simulink model "clonado_controlador"  (R2023b)
settings: Solver=ode45  StartTime=0.0  StopTime=10000  RelTol=1e-3
values from neighbouring files (symbols this model uses):
  D = 0    [control_pid_tuning.m]
libraries: neural x25, simulink x2, slpidlib x1
settings Model: Creator=q  LastModifiedBy=q

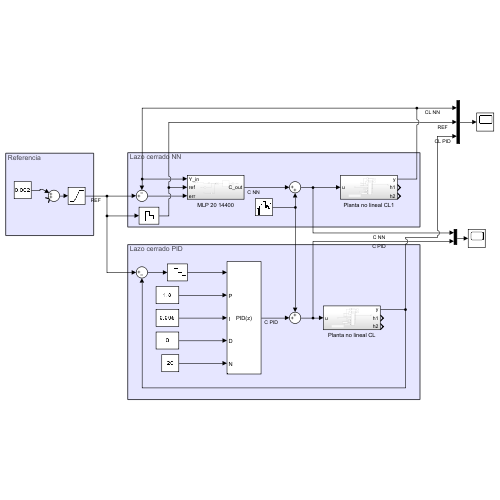
[thumbnail: Simulink's stored preview of the top-level diagram]
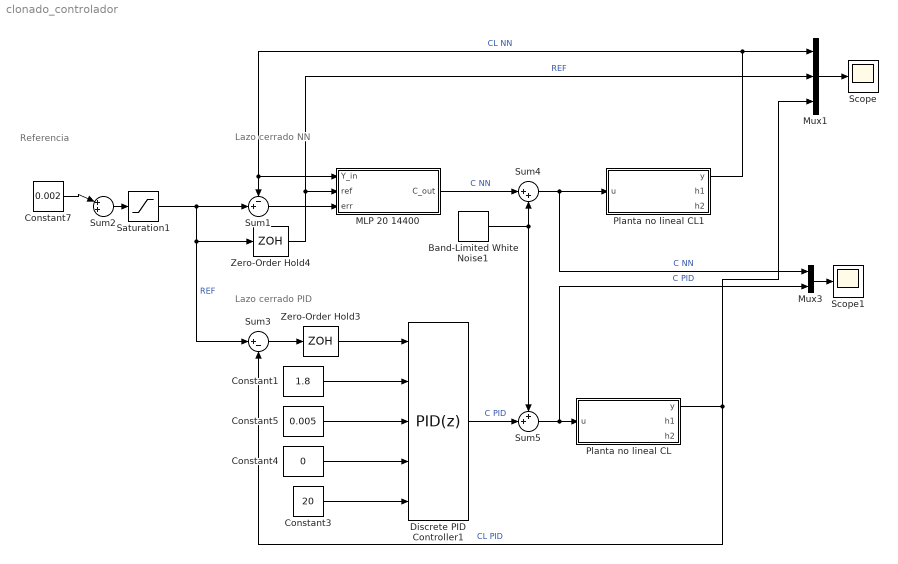
== system clonado_controlador ==
  note: Lazo cerrado NN
  note: Lazo cerrado PID
  note: Referencia
  Band-Limited White Noise1 : simulink/Sources/Band-Limited White Noise  Cov=[0.000002]  Ts=1500  seed=[23341]
  Constant1 : Constant  Value=1.8
  Constant3 : Constant  Value=20
  Constant4 : Constant  Value=0
  Constant5 : Constant  Value=0.005
  Constant7 : Constant  Value=0.002
  Discrete PID Controller1 : slpidlib/PID Controller  Controller=PID  Form=Parallel  TimeDomain=Discrete-time  UseExternalTs=off  SampleTime=-1  IntegratorMethod=Forward Euler  FilterMethod=Forward Euler  ControllerParametersSource=external  P=1  I=1  UseKiTs=off  D=0  N=100  UseFilter=on  TunerSelectOption=Transfer Function Based (PID Tuner App)  InitialConditionSource=internal  InitialConditionForIntegrator=0  InitialConditionForFilter=0  DifferentiatorICPrevScaledInput=0  ExternalReset=none  TrackingMode=off  Kt=1  LimitOutput=off  SatLimitsSource=internal  UpperSaturationLimit=inf  LowerSaturationLimit=-inf  LinearizeAsGain=off  AntiWindupMode=none  Kb=1  LimitIntegrator=off  UpperIntegratorSaturationLimit=inf  LowerIntegratorSaturationLimit=-inf  POutMin=[]  POutMax=[]  IOutMin=[]  IOutMax=[]  DOutMin=[]  DOutMax=[]  NOutMin=[]  NOutMax=[]  SumOutMin=[]  SumOutMax=[]  SaturationOutMin=[]  SaturationOutMax=[]  PParamMin=[]  PParamMax=[]  IParamMin=[]  IParamMax=[]  DParamMin=[]  DParamMax=[]  NParamMin=[]  NParamMax=[]  KbParamMin=[]  KbParamMax=[]  KtParamMin=[]  KtParamMax=[]  KbOutMin=[]  KbOutMax=[]  KtOutMin=[]  KtOutMax=[]  IntegratorOutMin=[]  IntegratorOutMax=[]  FilterOutMin=[]  FilterOutMax=[]  SumI1OutMin=[]  SumI1OutMax=[]  SumI2OutMin=[]  SumI2OutMax=[]  SumI3OutMin=[]  SumI3OutMax=[]  SumI4OutMin=[]  SumI4OutMax=[]  SumDOutMin=[]  SumDOutMax=[]  DifferentiatorOutMin=[]  DifferentiatorOutMax=[]  FilterDiffOutCoefMin=[]  FilterDiffOutCoefMax=[]  ReciprocalOutMin=[]  ReciprocalOutMax=[]  SumDenOutMin=[]  SumDenOutMax=[]  SumNumOutMin=[]  SumNumOutMax=[]  DivideOutMin=[]  DivideOutMax=[]  UdiffTsProdOutMin=[]  UdiffTsProdOutMax=[]  NTsProdOutMin=[]  NTsProdOutMax=[]  UintegralTsProdOutMin=[]  UintegralTsProdOutMax=[]  UngainTsProdOutMin=[]  UngainTsProdOutMax=[]  ClampingZeroOutDataTypeStr=Inherit: Inherit via back propagation  ClampingZeroOutMin=[]  ClampingZeroOutMax=[]  FilterDenConstantOutDataTypeStr=Inherit: Inherit via back propagation  FilterDenConstantOutMin=[]  FilterDenConstantOutMax=[]  PCopyOutDataTypeStr=Inherit: Inherit via back propagation  PCopyOutMin=[]  PCopyOutMax=[]  NCopyOutDataTypeStr=Inherit: Inherit via back propagation  NCopyOutMin=[]  NCopyOutMax=[]  IntegratorContinuousStateAttributes=''  IntegratorStateMustResolveToSignalObject=off  IntegratorRTWStateStorageClass=Auto  FilterContinuousStateAttributes=''  FilterStateMustResolveToSignalObject=off  FilterRTWStateStorageClass=Auto  ParallelPVariant=ExternalParameters  IdealPVariant=Disabled  IVariant=ExternalParameters  DVariant=ExternalParameters  IntegratorVariant=Discrete  SatVariant=Disabled  AWVariant=Passthrough  PCopyVariant=Disabled  TRVariant=Disabled  FdbkBlocksVariant=Forward  IdealPFdbkVariant=Disabled  SatFdbkVariant=Disabled  DerivativeFilterVariant=ForwardEulerFilter  NVariant=ExternalParameters  NCopyVariant=Disabled  FilterICVariant=InternalICsFilter  IntegratorICVariant=InternalICs  ExternalResetVariant=Disabled  TRSumVariant=Passthrough  SumFdbkVariant=Disabled  SumVariant=Sum_PID  TsampFilterVariant=InternalTs  TsampNgainVariant=Passthrough  TsampIntegralVariant=Disabled_SignalSpec  ExternalSaturationOutDataTypeStr=Inherit: Same as second input
      settings: LibrarySourceBlock=simulink/Discrete/Discrete PID Controller
  MLP 20 14400 : Subsystem
  Mux1 : Mux  Inputs=3
  Mux3 : Mux  Inputs=2
  Planta no lineal CL : Subsystem
  Planta no lineal CL1 : Subsystem
  Saturation1 : Saturate  UpperLimit=0.0022  LowerLimit=0.0018
  Scope : Scope
  Scope1 : Scope
  Sum1 : Sum  Inputs=-+|
  Sum2 : Sum  Inputs=|++|
  Sum3 : Sum  Inputs=|+-
  Sum4 : Sum  Inputs=|++
  Sum5 : Sum  Inputs=++|
  Zero-Order Hold3 : ZeroOrderHold
  Zero-Order Hold4 : ZeroOrderHold
  wires:
  Constant4/1 -> Discrete PID Controller1/4
  Constant3/1 -> Discrete PID Controller1/5
  Constant5/1 -> Discrete PID Controller1/3
  Constant1/1 -> Discrete PID Controller1/2
  Sum3/1 -> Zero-Order Hold3/1
  Planta no lineal CL/1(y) -> Sum3/2, Mux1/3  "CL PID"
  Zero-Order Hold3/1 -> Discrete PID Controller1/1
  Sum1/1 -> MLP 20 14400/3(err)
  Sum2/1 -> Saturation1/1
  Saturation1/1 -> Sum3/1, Zero-Order Hold4/1, Sum1/2  "REF"
  Planta no lineal CL1/1(y) -> Mux1/1, MLP 20 14400/1(Y_in), Sum1/1  "CL NN"
  Zero-Order Hold4/1 -> Mux1/2, MLP 20 14400/2(ref)  "REF"
  MLP 20 14400/1(C_out) -> Sum4/1  "C NN"
  Mux1/1 -> Scope/1
  Mux3/1 -> Scope1/1
  Constant7/1 -> Sum2/1
  Sum4/1 -> Mux3/1, Planta no lineal CL1/1(u)  "C NN"
  Band-Limited White Noise1/1 -> Sum5/1, Sum4/2
  Sum5/1 -> Mux3/2, Planta no lineal CL/1(u)  "C PID"
  Discrete PID Controller1/1 -> Sum5/2  "C PID"

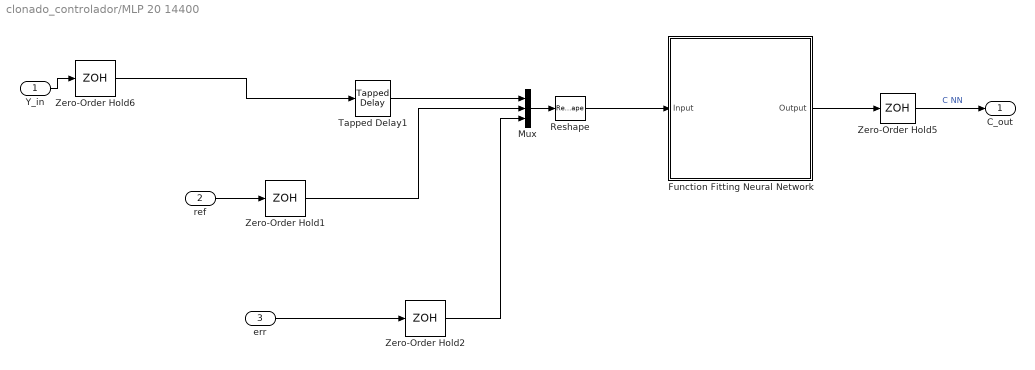
== system clonado_controlador/MLP 20 14400 ==
  Y_in : Inport
  ref : Inport  Port=2
  err : Inport  Port=3
  Function Fitting Neural Network : Subsystem
      mask help: Function Fitting Neural Network
      mask Display: e = 0.06;c1 = [120 150 230]/255;c2 = ([120 150 230]+0)/383;c3 = ([120 150 230]+128)/383;patch([0 1 1 0],[0 0 1 1],c1);patch([0 1 1 1-e 1-e 0+e],[0 0 1 1-e 0+e 0+e],c2);patch([0 0 1 1-e 0+e 0+e],[0 1 1 1-e 1-e 0+e],c3);plot([0 1 1 0 0],[0 0 1 1 0]);fprintf('NNET');port_label('input',1,' Input');port_label('output',1,'Output ');
  Mux : Mux  Inputs=3
  Reshape : Reshape  OutputDimensionality=Column vector (2-D)
  Tapped Delay1 : simulink/Discrete/Tapped Delay  vinit=0  samptime=1  NumDelays=10  DelayOrder=Newest  includeCurrent=off
  Zero-Order Hold{1..2,5..6} (4 alike) : ZeroOrderHold
  C_out : Outport
  wires:
  Mux/1 -> Reshape/1
  Tapped Delay1/1 -> Mux/1
  Reshape/1 -> Function Fitting Neural Network/1(Input)
  Y_in/1 -> Zero-Order Hold6/1
  ref/1 -> Zero-Order Hold1/1
  err/1 -> Zero-Order Hold2/1
  Function Fitting Neural Network/1(Output) -> Zero-Order Hold5/1
  Zero-Order Hold6/1 -> Tapped Delay1/1
  Zero-Order Hold1/1 -> Mux/2
  Zero-Order Hold2/1 -> Mux/3
  Zero-Order Hold5/1 -> C_out/1  "C NN"

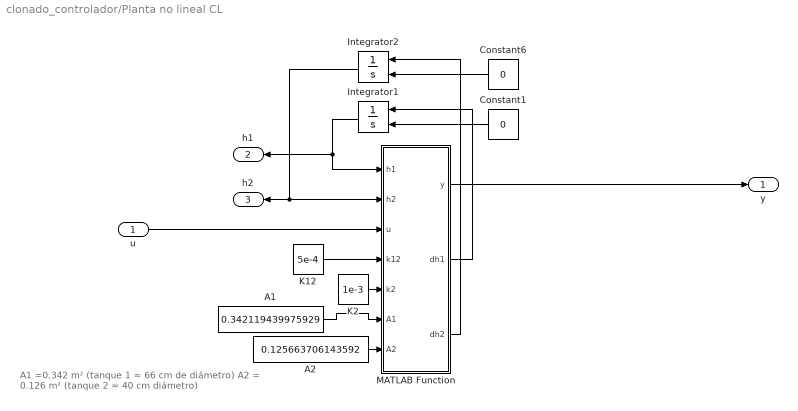
== system clonado_controlador/Planta no lineal CL ==
  note: A1 =0.342   m²   (tanque 1 ≈ 66 cm de diámetro)
      | A2 = 0.126   m²   (tanque 2 ≈ 40 cm diámetro)
  u : Inport
  A1 : Constant  Value=0.342119439975929
  A2 : Constant  Value=0.125663706143592
  Constant1 : Constant  Value=0
  Constant6 : Constant  Value=0
  Integrator1 : Integrator  InitialConditionSource=external
  Integrator2 : Integrator  InitialConditionSource=external
  K12 : Constant  Value=5e-4
  K2 : Constant  Value=1e-3
  MATLAB Function : MATLAB Function  TreatAsAtomicUnit=on
  y : Outport
  h1 : Outport  Port=2
  h2 : Outport  Port=3
  wires:
  K2/1 -> MATLAB Function/5(k2)
  MATLAB Function/3(dh2) -> Integrator2/1
  MATLAB Function/2(dh1) -> Integrator1/1
  Integrator1/1 -> h1/1, MATLAB Function/1(h1)
  Constant6/1 -> Integrator2/2
  A2/1 -> MATLAB Function/7(A2)
  Constant1/1 -> Integrator1/2
  u/1 -> MATLAB Function/3(u)
  MATLAB Function/1(y) -> y/1
  Integrator2/1 -> h2/1, MATLAB Function/2(h2)
  A1/1 -> MATLAB Function/6(A1)
  K12/1 -> MATLAB Function/4(k12)

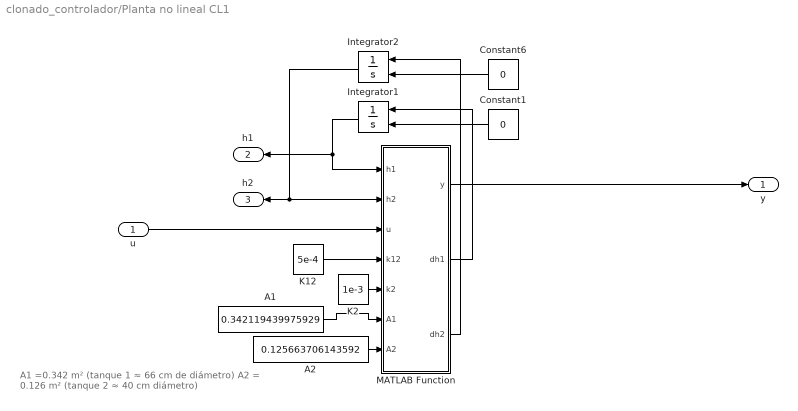
== system clonado_controlador/Planta no lineal CL1 ==
  note: A1 =0.342   m²   (tanque 1 ≈ 66 cm de diámetro)
      | A2 = 0.126   m²   (tanque 2 ≈ 40 cm diámetro)
  u : Inport
  A1 : Constant  Value=0.342119439975929
  A2 : Constant  Value=0.125663706143592
  Constant1 : Constant  Value=0
  Constant6 : Constant  Value=0
  Integrator1 : Integrator  InitialConditionSource=external
  Integrator2 : Integrator  InitialConditionSource=external
  K12 : Constant  Value=5e-4
  K2 : Constant  Value=1e-3
  MATLAB Function : MATLAB Function  TreatAsAtomicUnit=on
  y : Outport
  h1 : Outport  Port=2
  h2 : Outport  Port=3
  wires:
  K12/1 -> MATLAB Function/4(k12)
  A1/1 -> MATLAB Function/6(A1)
  Integrator2/1 -> MATLAB Function/2(h2), h2/1
  MATLAB Function/1(y) -> y/1
  u/1 -> MATLAB Function/3(u)
  Constant1/1 -> Integrator1/2
  A2/1 -> MATLAB Function/7(A2)
  Constant6/1 -> Integrator2/2
  Integrator1/1 -> MATLAB Function/1(h1), h1/1
  MATLAB Function/2(dh1) -> Integrator1/1
  MATLAB Function/3(dh2) -> Integrator2/1
  K2/1 -> MATLAB Function/5(k2)

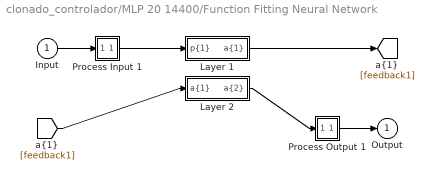
== system clonado_controlador/MLP 20 14400/Function Fitting Neural Network ==
  Input : Inport  PortDimensions=12
      mask Display: e = 0.06;c1 = [120 230 180]/255;c2 = ([120 230 180]+0)/(256+128);c3 = ([120 230 180]+128)/(256+128);patch([0 1 1 0],[0 0 1 1],c1);patch([0 1 1 1-e 1-e 0+e],[0 0 1 1-e 0+e 0+e],c2);patch([0 0 1 1-e 0+e 0+e],[0 1 1 1-e 1-e 0+e],c3);plot([0 1 1 0 0],[0 0 1 1 0]);
  Layer 1 : Subsystem
      mask Display: e = 0.06;c1 = [120 150 230]/255;c2 = ([120 150 230]+0)/383;c3 = ([120 150 230]+128)/383;patch([0 1 1 0],[0 0 1 1],c1);patch([0 1 1 1-e 1-e 0+e],[0 0 1 1-e 0+e 0+e],c2);patch([0 0 1 1-e 0+e 0+e],[0 1 1 1-e 1-e 0+e],c3);plot([0 1 1 0 0],[0 0 1 1 0]);
  Layer 2 : Subsystem
      mask Display: e = 0.06;c1 = [120 150 230]/255;c2 = ([120 150 230]+0)/383;c3 = ([120 150 230]+128)/383;patch([0 1 1 0],[0 0 1 1],c1);patch([0 1 1 1-e 1-e 0+e],[0 0 1 1-e 0+e 0+e],c2);patch([0 0 1 1-e 0+e 0+e],[0 1 1 1-e 1-e 0+e],c3);plot([0 1 1 0 0],[0 0 1 1 0]);
  Process Input 1 : Subsystem
      mask Display: e = 0.06;c1 = [120 150 230]/255;c2 = ([120 150 230]+0)/383;c3 = ([120 150 230]+128)/383;patch([0 1 1 0],[0 0 1 1],c1);patch([0 1 1 1-e 1-e 0+e],[0 0 1 1-e 0+e 0+e],c2);patch([0 0 1 1-e 0+e 0+e],[0 1 1 1-e 1-e 0+e],c3);plot([0 1 1 0 0],[0 0 1 1 0]);
  Process Output 1 : Subsystem
      mask Display: e = 0.06;c1 = [120 150 230]/255;c2 = ([120 150 230]+0)/383;c3 = ([120 150 230]+128)/383;patch([0 1 1 0],[0 0 1 1],c1);patch([0 1 1 1-e 1-e 0+e],[0 0 1 1-e 0+e 0+e],c2);patch([0 0 1 1-e 0+e 0+e],[0 1 1 1-e 1-e 0+e],c3);plot([0 1 1 0 0],[0 0 1 1 0]);
  Output : Outport  InitialOutput=0
      mask Display: e = 0.06;c1 = [120 230 180]/255;c2 = ([120 230 180]+0)/(256+128);c3 = ([120 230 180]+128)/(256+128);patch([0 1 1 0],[0 0 1 1],c1);patch([0 1 1 1-e 1-e 0+e],[0 0 1 1-e 0+e 0+e],c2);patch([0 0 1 1-e 0+e 0+e],[0 1 1 1-e 1-e 0+e],c3);plot([0 1 1 0 0],[0 0 1 1 0]);
  wires:
  Input/1 -> Process Input 1/1(x)
  Process Output 1/1(y) -> Output/1
  Process Input 1/1(p) -> Layer 1/1("p{1}")
  Layer 1/1("a{1}") -> [feedback1]
  [feedback1] -> Layer 2/1("a{1} ")
  Layer 2/1("a{2}") -> Process Output 1/1(a)

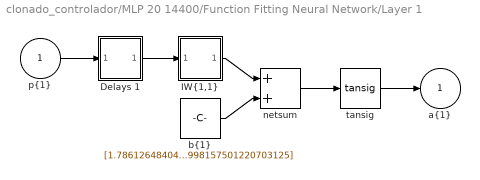
== system clonado_controlador/MLP 20 14400/Function Fitting Neural Network/Layer 1 ==
  "p{1}" : Inport  PortDimensions=12
      mask Display: e = 0.06;c1 = [120 230 180]/255;c2 = ([120 230 180]+0)/(256+128);c3 = ([120 230 180]+128)/(256+128);patch([0 1 1 0],[0 0 1 1],c1);patch([0 1 1 1-e 1-e 0+e],[0 0 1 1-e 0+e 0+e],c2);patch([0 0 1 1-e 0+e 0+e],[0 1 1 1-e 1-e 0+e],c3);plot([0 1 1 0 0],[0 0 1 1 0]);
  Delays 1 : Subsystem
      mask Display: e = 0.06;c1 = [120 150 230]/255;c2 = ([120 150 230]+0)/383;c3 = ([120 150 230]+128)/383;patch([0 1 1 0],[0 0 1 1],c1);patch([0 1 1 1-e 1-e 0+e],[0 0 1 1-e 0+e 0+e],c2);patch([0 0 1 1-e 0+e 0+e],[0 1 1 1-e 1-e 0+e],c3);plot([0 1 1 0 0],[0 0 1 1 0]);disp('0');
  "IW{1,1}" : Subsystem
      mask Display: e = 0.06;c1 = [120 150 230]/255;c2 = ([120 150 230]+0)/383;c3 = ([120 150 230]+128)/383;patch([0 1 1 0],[0 0 1 1],c1);patch([0 1 1 1-e 1-e 0+e],[0 0 1 1-e 0+e 0+e],c2);patch([0 0 1 1-e 0+e 0+e],[0 1 1 1-e 1-e 0+e],c3);plot([0 1 1 0 0],[0 0 1 1 0]);disp('W');
  "b{1}" : Constant  Value=[1.7861264840469488479612891751457937061786651611328125;-1.61568698376680064399124603369273245334625244140625;1.3995470416459114826324139357893727719783782958984375;-1.405995168242849313600117966416291892528533935546875;1.0865257979502944696292843218543566763401031494140625;-0.77998085491395519053270390941179357469081878662109375;-0.622862839542821067340128138312138617038726806640625;-0.71522848151096762858713873356464318931102752685546875;-0.25889837816397232028720054586301557719707489013671875;-0.04969359609535091426568698125265655107796192169189453125;-0.053671914504017238789490562567152664996683597564697265625;-0.26459524720328742031227875486365519464015960693359375;-0.58446847806037471872997457467135973274707794189453125;-0.80707695263700018895036691901623271405696868896484375;1.4965041243393375491876895466702990233898162841796875;-1.027860752504613284230572389787994325160980224609375;1.3992942558582941448008796214708127081394195556640625;1.39170148730409071191616021678782999515533447265625;-1.644863122293897195191902937949635088443756103515625;1.724716661469497314129739606869406998157501220703125]
      mask Display: e = 0.06;c1 = [120 150 230]/255;c2 = ([120 150 230]+0)/383;c3 = ([120 150 230]+128)/383;patch([0 1 1 0],[0 0 1 1],c1);patch([0 1 1 1-e 1-e 0+e],[0 0 1 1-e 0+e 0+e],c2);patch([0 0 1 1-e 0+e 0+e],[0 1 1 1-e 1-e 0+e],c3);plot([0 1 1 0 0],[0 0 1 1 0]);disp('b');
  netsum : Sum  Inputs=2  InputSameDT=on  SaturateOnIntegerOverflow=on  OutDataTypeStr=Inherit: Same as first input
      mask Display: e = 0.06;c1 = [120 150 230]/255;c2 = ([120 150 230]+0)/383;c3 = ([120 150 230]+128)/383;patch([0 1 1 0],[0 0 1 1],c1);patch([0 1 1 1-e 1-e 0+e],[0 0 1 1-e 0+e 0+e],c2);patch([0 0 1 1-e 0+e 0+e],[0 1 1 1-e 1-e 0+e],c3);plot([0 1 1 0 0],[0 0 1 1 0]);disp('+');
  tansig : neural/Transfer Functions/tansig
  "a{1}" : Outport  InitialOutput=[0;0;0;0;0;0;0;0;0;0;0;0;0;0;0;0;0;0;0;0]
      mask Display: e = 0.06;c1 = [120 230 180]/255;c2 = ([120 230 180]+0)/(256+128);c3 = ([120 230 180]+128)/(256+128);patch([0 1 1 0],[0 0 1 1],c1);patch([0 1 1 1-e 1-e 0+e],[0 0 1 1-e 0+e 0+e],c2);patch([0 0 1 1-e 0+e 0+e],[0 1 1 1-e 1-e 0+e],c3);plot([0 1 1 0 0],[0 0 1 1 0]);
  wires:
  "p{1}"/1 -> Delays 1/1("p{1}")
  Delays 1/1("pd{1,1}") -> "IW{1,1}"/1("pd{1,1}")
  "IW{1,1}"/1("iz{1,1}") -> netsum/1
  "b{1}"/1 -> netsum/2
  netsum/1 -> tansig/1
  tansig/1 -> "a{1}"/1

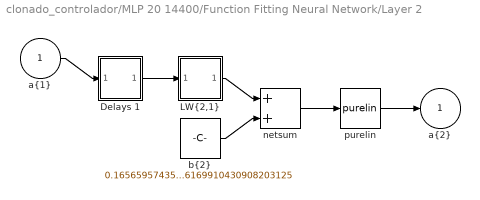
== system clonado_controlador/MLP 20 14400/Function Fitting Neural Network/Layer 2 ==
  "a{1} " : Inport  PortDimensions=20
      mask Display: e = 0.06;c1 = [120 230 180]/255;c2 = ([120 230 180]+0)/(256+128);c3 = ([120 230 180]+128)/(256+128);patch([0 1 1 0],[0 0 1 1],c1);patch([0 1 1 1-e 1-e 0+e],[0 0 1 1-e 0+e 0+e],c2);patch([0 0 1 1-e 0+e 0+e],[0 1 1 1-e 1-e 0+e],c3);plot([0 1 1 0 0],[0 0 1 1 0]);
  Delays 1 : Subsystem
      mask Display: e = 0.06;c1 = [120 150 230]/255;c2 = ([120 150 230]+0)/383;c3 = ([120 150 230]+128)/383;patch([0 1 1 0],[0 0 1 1],c1);patch([0 1 1 1-e 1-e 0+e],[0 0 1 1-e 0+e 0+e],c2);patch([0 0 1 1-e 0+e 0+e],[0 1 1 1-e 1-e 0+e],c3);plot([0 1 1 0 0],[0 0 1 1 0]);disp('0');
  "LW{2,1}" : Subsystem
      mask Display: e = 0.06;c1 = [120 150 230]/255;c2 = ([120 150 230]+0)/383;c3 = ([120 150 230]+128)/383;patch([0 1 1 0],[0 0 1 1],c1);patch([0 1 1 1-e 1-e 0+e],[0 0 1 1-e 0+e 0+e],c2);patch([0 0 1 1-e 0+e 0+e],[0 1 1 1-e 1-e 0+e],c3);plot([0 1 1 0 0],[0 0 1 1 0]);disp('W');
  "b{2}" : Constant  Value=0.1656595743509694795836395542210084386169910430908203125
      mask Display: e = 0.06;c1 = [120 150 230]/255;c2 = ([120 150 230]+0)/383;c3 = ([120 150 230]+128)/383;patch([0 1 1 0],[0 0 1 1],c1);patch([0 1 1 1-e 1-e 0+e],[0 0 1 1-e 0+e 0+e],c2);patch([0 0 1 1-e 0+e 0+e],[0 1 1 1-e 1-e 0+e],c3);plot([0 1 1 0 0],[0 0 1 1 0]);disp('b');
  netsum : Sum  Inputs=2  InputSameDT=on  SaturateOnIntegerOverflow=on  OutDataTypeStr=Inherit: Same as first input
      mask Display: e = 0.06;c1 = [120 150 230]/255;c2 = ([120 150 230]+0)/383;c3 = ([120 150 230]+128)/383;patch([0 1 1 0],[0 0 1 1],c1);patch([0 1 1 1-e 1-e 0+e],[0 0 1 1-e 0+e 0+e],c2);patch([0 0 1 1-e 0+e 0+e],[0 1 1 1-e 1-e 0+e],c3);plot([0 1 1 0 0],[0 0 1 1 0]);disp('+');
  purelin : neural/Transfer Functions/purelin
  "a{2}" : Outport  InitialOutput=0
      mask Display: e = 0.06;c1 = [120 230 180]/255;c2 = ([120 230 180]+0)/(256+128);c3 = ([120 230 180]+128)/(256+128);patch([0 1 1 0],[0 0 1 1],c1);patch([0 1 1 1-e 1-e 0+e],[0 0 1 1-e 0+e 0+e],c2);patch([0 0 1 1-e 0+e 0+e],[0 1 1 1-e 1-e 0+e],c3);plot([0 1 1 0 0],[0 0 1 1 0]);
  wires:
  "a{1} "/1 -> Delays 1/1("p{2}")
  Delays 1/1("pd{2,1}") -> "LW{2,1}"/1("ad{2,1}")
  "LW{2,1}"/1("lz{2,1}") -> netsum/1
  "b{2}"/1 -> netsum/2
  netsum/1 -> purelin/1
  purelin/1 -> "a{2}"/1

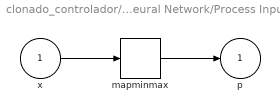
== system clonado_controlador/MLP 20 14400/Function Fitting Neural Network/Process Input 1 ==
  x : Inport  PortDimensions=12
      mask Display: e = 0.06;c1 = [120 230 180]/255;c2 = ([120 230 180]+0)/(256+128);c3 = ([120 230 180]+128)/(256+128);patch([0 1 1 0],[0 0 1 1],c1);patch([0 1 1 1-e 1-e 0+e],[0 0 1 1-e 0+e 0+e],c2);patch([0 0 1 1-e 0+e 0+e],[0 1 1 1-e 1-e 0+e],c3);plot([0 1 1 0 0],[0 0 1 1 0]);
  mapminmax : neural/Processing Functions/mapminmax  xmin=[0.000424806409659916027476977973265;0.000397996685492861058171948362983;0.000369232373214941473043432251799;0.000338129690514188906407672119414;0.000304153140997853515745119601377;0.000266510837110306929818859256187;0.000223929080485324612497660679011;0.000174065778287826162205875757394;0.000111358850198966946869368055406;0;0.00195886511982748968280221291138;-0.000139017162043636715446082163794]  xmax=[0.00210067175776176232743219784993;0.00210067175776176232743219784993;0.00210067175776176232743219784993;0.00210067175776176232743219784993;0.00210067175776176232743219784993;0.00210067175776176232743219784993;0.00210067175776176232743219784993;0.00210067175776176232743219784993;0.00210067175776176232743219784993;0.00210067175776176232743219784993;0.00210673473128668905379745623918;0.00156599539225801571290519476065]  ymin=-1  ymax=1
  p : Outport  PortDimensions=12
      mask Display: e = 0.06;c1 = [120 230 180]/255;c2 = ([120 230 180]+0)/(256+128);c3 = ([120 230 180]+128)/(256+128);patch([0 1 1 0],[0 0 1 1],c1);patch([0 1 1 1-e 1-e 0+e],[0 0 1 1-e 0+e 0+e],c2);patch([0 0 1 1-e 0+e 0+e],[0 1 1 1-e 1-e 0+e],c3);plot([0 1 1 0 0],[0 0 1 1 0]);
  wires:
  x/1 -> mapminmax/1
  mapminmax/1 -> p/1

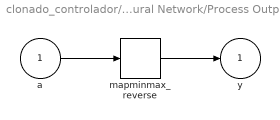
== system clonado_controlador/MLP 20 14400/Function Fitting Neural Network/Process Output 1 ==
  a : Inport  PortDimensions=1
      mask Display: e = 0.06;c1 = [120 230 180]/255;c2 = ([120 230 180]+0)/(256+128);c3 = ([120 230 180]+128)/(256+128);patch([0 1 1 0],[0 0 1 1],c1);patch([0 1 1 1-e 1-e 0+e],[0 0 1 1-e 0+e 0+e],c2);patch([0 0 1 1-e 0+e 0+e],[0 1 1 1-e 1-e 0+e],c3);plot([0 1 1 0 0],[0 0 1 1 0]);
  mapminmax_reverse : neural/Processing Functions/mapminmax_reverse  xmin=0.00184065834880211848939568497485  xmax=0.00290653799161805182979523287656  ymin=-1  ymax=1
  y : Outport  PortDimensions=1
      mask Display: e = 0.06;c1 = [120 230 180]/255;c2 = ([120 230 180]+0)/(256+128);c3 = ([120 230 180]+128)/(256+128);patch([0 1 1 0],[0 0 1 1],c1);patch([0 1 1 1-e 1-e 0+e],[0 0 1 1-e 0+e 0+e],c2);patch([0 0 1 1-e 0+e 0+e],[0 1 1 1-e 1-e 0+e],c3);plot([0 1 1 0 0],[0 0 1 1 0]);
  wires:
  a/1 -> mapminmax_reverse/1
  mapminmax_reverse/1 -> y/1

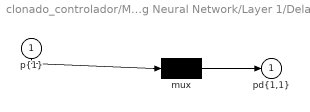
== system clonado_controlador/MLP 20 14400/Function Fitting Neural Network/Layer 1/Delays 1 ==
  "p{1}" : Inport  PortDimensions=12
      mask Display: e = 0.06;c1 = [120 230 180]/255;c2 = ([120 230 180]+0)/(256+128);c3 = ([120 230 180]+128)/(256+128);patch([0 1 1 0],[0 0 1 1],c1);patch([0 1 1 1-e 1-e 0+e],[0 0 1 1-e 0+e 0+e],c2);patch([0 0 1 1-e 0+e 0+e],[0 1 1 1-e 1-e 0+e],c3);plot([0 1 1 0 0],[0 0 1 1 0]);
  mux : Mux  Inputs=1
      mask Display: e = 0.06;c1 = [120 150 230]/255;c2 = ([120 150 230]+0)/383;c3 = ([120 150 230]+128)/383;patch([0 1 1 0],[0 0 1 1],c1);patch([0 1 1 1-e 1-e 0+e],[0 0 1 1-e 0+e 0+e],c2);patch([0 0 1 1-e 0+e 0+e],[0 1 1 1-e 1-e 0+e],c3);plot([0 1 1 0 0],[0 0 1 1 0]);disp('Mux')
  "pd{1,1}" : Outport
      mask Display: e = 0.06;c1 = [120 230 180]/255;c2 = ([120 230 180]+0)/(256+128);c3 = ([120 230 180]+128)/(256+128);patch([0 1 1 0],[0 0 1 1],c1);patch([0 1 1 1-e 1-e 0+e],[0 0 1 1-e 0+e 0+e],c2);patch([0 0 1 1-e 0+e 0+e],[0 1 1 1-e 1-e 0+e],c3);plot([0 1 1 0 0],[0 0 1 1 0]);
  wires:
  "p{1}"/1 -> mux/1
  mux/1 -> "pd{1,1}"/1

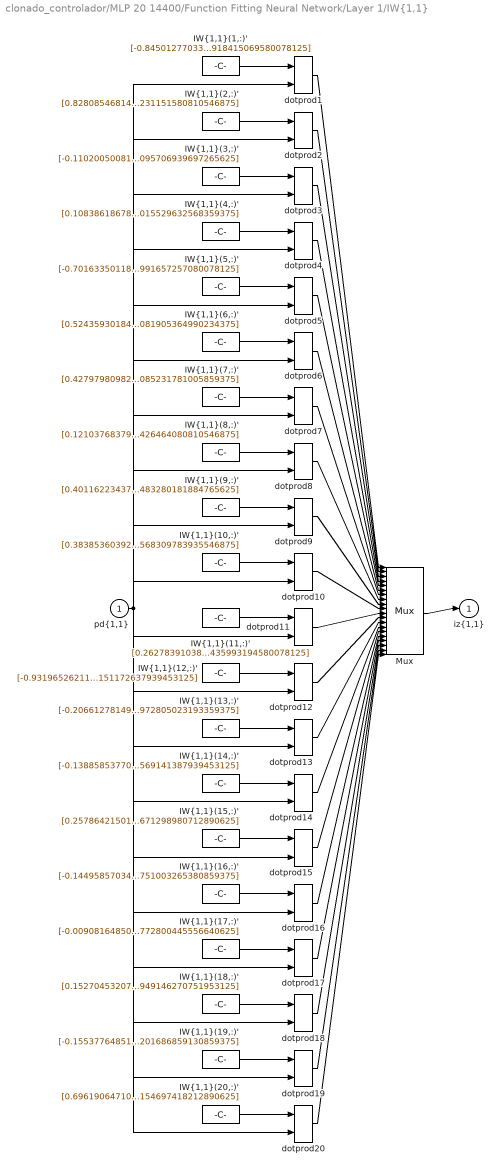
== system clonado_controlador/MLP 20 14400/Function Fitting Neural Network/Layer 1/IW{1,1} ==
  "pd{1,1}" : Inport  PortDimensions=12
      mask Display: e = 0.06;c1 = [120 230 180]/255;c2 = ([120 230 180]+0)/(256+128);c3 = ([120 230 180]+128)/(256+128);patch([0 1 1 0],[0 0 1 1],c1);patch([0 1 1 1-e 1-e 0+e],[0 0 1 1-e 0+e 0+e],c2);patch([0 0 1 1-e 0+e 0+e],[0 1 1 1-e 1-e 0+e],c3);plot([0 1 1 0 0],[0 0 1 1 0]);
  "IW{1,1}(1,:)'" : Constant  Value=[-0.845012770332619567170695518143475055694580078125;0.07732932948601527189946835960654425434768199920654296875;-0.041359218778451618814262502610290539450943470001220703125;0.57208430831804835126064290307112969458103179931640625;0.0819798649305745474880069423306849785149097442626953125;0.11968658736390237751212595185279496945440769195556640625;0.294815667220991783903372152053634636104106903076171875;0.845972951520416405202240639482624828815460205078125;0.733023615958870333741970171104185283184051513671875;0.810267793286779891559490351937711238861083984375;-0.2252103705837339708839550667107687331736087799072265625;-0.163662973267360734030972935215686447918415069580078125]
      mask Display: e = 0.06;c1 = [120 150 230]/255;c2 = ([120 150 230]+0)/383;c3 = ([120 150 230]+128)/383;patch([0 1 1 0],[0 0 1 1],c1);patch([0 1 1 1-e 1-e 0+e],[0 0 1 1-e 0+e 0+e],c2);patch([0 0 1 1-e 0+e 0+e],[0 1 1 1-e 1-e 0+e],c3);plot([0 1 1 0 0],[0 0 1 1 0]);disp('Weights');
  "IW{1,1}(10,:)'" : Constant  Value=[0.383853603928103359610446432270691730082035064697265625;0.9561315668646894749826969928108155727386474609375;0.282312644026379067074827844407991506159305572509765625;-0.271380093607639538699771719620912335813045501708984375;0.07611725353725772025281770538640557788312435150146484375;-0.1543612068514981505717997833926347084343433380126953125;-0.9914220353297553689486676375963725149631500244140625;0.85334016411793822687315014263731427490711212158203125;0.008452359785290609883734447294045821763575077056884765625;-0.303281605793638942003553893300704658031463623046875;0.37761369653873810836586244477075524628162384033203125;0.11169007743695973100539475808545830659568309783935546875]
      mask Display: e = 0.06;c1 = [120 150 230]/255;c2 = ([120 150 230]+0)/383;c3 = ([120 150 230]+128)/383;patch([0 1 1 0],[0 0 1 1],c1);patch([0 1 1 1-e 1-e 0+e],[0 0 1 1-e 0+e 0+e],c2);patch([0 0 1 1-e 0+e 0+e],[0 1 1 1-e 1-e 0+e],c3);plot([0 1 1 0 0],[0 0 1 1 0]);disp('Weights');
  "IW{1,1}(11,:)'" : Constant  Value=[0.26278391038896520282008850699639879167079925537109375;-0.39416983006497841035553619803977198898792266845703125;0.85040624443631329665294060760061256587505340576171875;0.56883755072459629698045091572566889226436614990234375;-0.6512073295448643772687091768602840602397918701171875;0.2748033253508086470873195139574818313121795654296875;-0.570426851016609948175073441234417259693145751953125;0.69054308552530108133993280716822482645511627197265625;0.7062957529674929180174558496219106018543243408203125;0.2365464524023907222360918467529700137674808502197265625;0.303535818481531716184207425612839870154857635498046875;-0.498922885967328533229903086976264603435993194580078125]
      mask Display: e = 0.06;c1 = [120 150 230]/255;c2 = ([120 150 230]+0)/383;c3 = ([120 150 230]+128)/383;patch([0 1 1 0],[0 0 1 1],c1);patch([0 1 1 1-e 1-e 0+e],[0 0 1 1-e 0+e 0+e],c2);patch([0 0 1 1-e 0+e 0+e],[0 1 1 1-e 1-e 0+e],c3);plot([0 1 1 0 0],[0 0 1 1 0]);disp('Weights');
  "IW{1,1}(12,:)'" : Constant  Value=[-0.931965262115012738064478980959393084049224853515625;0.61260477904368049184569144927081651985645294189453125;-0.25544213188489173216311201031203381717205047607421875;0.87867114839822868521679311015759594738483428955078125;-0.003958964330272305744140570737954476498998701572418212890625;0.211215984403561041204966386430896818637847900390625;0.6337174601243484861612387248896993696689605712890625;0.332675761685613247120585356242372654378414154052734375;0.50894519197491894235696463510976172983646392822265625;-0.1440798689523048736749188947214861400425434112548828125;0.09554437465149935582164886227474198676645755767822265625;-0.53328571096418120323079392619547434151172637939453125]
      mask Display: e = 0.06;c1 = [120 150 230]/255;c2 = ([120 150 230]+0)/383;c3 = ([120 150 230]+128)/383;patch([0 1 1 0],[0 0 1 1],c1);patch([0 1 1 1-e 1-e 0+e],[0 0 1 1-e 0+e 0+e],c2);patch([0 0 1 1-e 0+e 0+e],[0 1 1 1-e 1-e 0+e],c3);plot([0 1 1 0 0],[0 0 1 1 0]);disp('Weights');
  "IW{1,1}(13,:)'" : Constant  Value=[-0.20661278149948270055347165907733142375946044921875;-0.928666659200457100808989707729779183864593505859375;-0.446874876311327773326098622419522143900394439697265625;-0.274042451254566277185631406609900295734405517578125;-0.5563730514213898192821261545759625732898712158203125;-0.3830619554637630930216118940734304487705230712890625;0.1444155330533601622189365798476501367986202239990234375;-0.490606264625608134988254960262565873563289642333984375;0.8492931457697785457838790534879080951213836669921875;-0.1515125820259310140958319834680878557264804840087890625;0.0784100086265687445941097166723920963704586029052734375;-0.64635234670450980587474987260065972805023193359375]
      mask Display: e = 0.06;c1 = [120 150 230]/255;c2 = ([120 150 230]+0)/383;c3 = ([120 150 230]+128)/383;patch([0 1 1 0],[0 0 1 1],c1);patch([0 1 1 1-e 1-e 0+e],[0 0 1 1-e 0+e 0+e],c2);patch([0 0 1 1-e 0+e 0+e],[0 1 1 1-e 1-e 0+e],c3);plot([0 1 1 0 0],[0 0 1 1 0]);disp('Weights');
  "IW{1,1}(14,:)'" : Constant  Value=[-0.1388585377078282723228852546526468358933925628662109375;-0.7464929933156547736672337123309262096881866455078125;-0.034512860743560906662263931821144069544970989227294921875;-0.95590163032006592036537995227263309061527252197265625;-0.00288480688347894122236514391488526598550379276275634765625;0.62971268798649482345552996775950305163860321044921875;0.496062649680631351234438852770836092531681060791015625;-0.517115677284845087768871962907724082469940185546875;0.66452788803303752818152361214742995798587799072265625;-0.42264701904070756111053697168244980275630950927734375;-0.1996409257339550047394283183166407980024814605712890625;0.1003436688399668430538014263220247812569141387939453125]
      mask Display: e = 0.06;c1 = [120 150 230]/255;c2 = ([120 150 230]+0)/383;c3 = ([120 150 230]+128)/383;patch([0 1 1 0],[0 0 1 1],c1);patch([0 1 1 1-e 1-e 0+e],[0 0 1 1-e 0+e 0+e],c2);patch([0 0 1 1-e 0+e 0+e],[0 1 1 1-e 1-e 0+e],c3);plot([0 1 1 0 0],[0 0 1 1 0]);disp('Weights');
  "IW{1,1}(15,:)'" : Constant  Value=[0.257864215013866304726519729229039512574672698974609375;-0.67714604805208267190863580253790132701396942138671875;-0.80026635753082786539636117595364339649677276611328125;-0.94825070055116855716192958425381220877170562744140625;0.2506350965035151201476537607959471642971038818359375;-0.249664875319993651014982560809585265815258026123046875;-0.5235777620627881656645286057027988135814666748046875;0.100444211398857119466043741340399719774723052978515625;-0.068840486471667461376711116827209480106830596923828125;0.83049950973557196132190938442363403737545013427734375;0.0849727846666509523121391111999400891363620758056640625;0.7727501127090088406390577802085317671298980712890625]
      mask Display: e = 0.06;c1 = [120 150 230]/255;c2 = ([120 150 230]+0)/383;c3 = ([120 150 230]+128)/383;patch([0 1 1 0],[0 0 1 1],c1);patch([0 1 1 1-e 1-e 0+e],[0 0 1 1-e 0+e 0+e],c2);patch([0 0 1 1-e 0+e 0+e],[0 1 1 1-e 1-e 0+e],c3);plot([0 1 1 0 0],[0 0 1 1 0]);disp('Weights');
  "IW{1,1}(16,:)'" : Constant  Value=[-0.1449585703471254760632547231580247171223163604736328125;0.6748777379211059468389066751115024089813232421875;-0.2189257627018742213831359322284697555005550384521484375;0.55547820053578511600989031649078242480754852294921875;-0.705964621490989596708232056698761880397796630859375;0.76841323335674693861818695950205437839031219482421875;-0.76302308965427700915284958682605065405368804931640625;-0.163997518526094399060610840024310164153575897216796875;-0.41238308652295774248131010608631186187267303466796875;0.293908807940316207929498659723321907222270965576171875;0.39015738974396974025893314319546334445476531982421875;0.55399804857473267105660852394066751003265380859375]
      mask Display: e = 0.06;c1 = [120 150 230]/255;c2 = ([120 150 230]+0)/383;c3 = ([120 150 230]+128)/383;patch([0 1 1 0],[0 0 1 1],c1);patch([0 1 1 1-e 1-e 0+e],[0 0 1 1-e 0+e 0+e],c2);patch([0 0 1 1-e 0+e 0+e],[0 1 1 1-e 1-e 0+e],c3);plot([0 1 1 0 0],[0 0 1 1 0]);disp('Weights');
  "IW{1,1}(17,:)'" : Constant  Value=[-0.0090816485071997000988464066040251054801046848297119140625;-0.018520935425686231579067708707952988334000110626220703125;0.382175740181092515879157645031227730214595794677734375;0.64460016943107856235428698710165917873382568359375;0.50631963181918460126240688623511232435703277587890625;-0.60600982114890289409459001035429537296295166015625;-0.74910811083996498016546183862374164164066314697265625;0.334947808962641868646414877730421721935272216796875;-0.8326586837199745350091006912407465279102325439453125;-0.759168801725680797432005419977940618991851806640625;-0.0951116173114518737019551508637960068881511688232421875;0.37320898184212725201547300457605160772800445556640625]
      mask Display: e = 0.06;c1 = [120 150 230]/255;c2 = ([120 150 230]+0)/383;c3 = ([120 150 230]+128)/383;patch([0 1 1 0],[0 0 1 1],c1);patch([0 1 1 1-e 1-e 0+e],[0 0 1 1-e 0+e 0+e],c2);patch([0 0 1 1-e 0+e 0+e],[0 1 1 1-e 1-e 0+e],c3);plot([0 1 1 0 0],[0 0 1 1 0]);disp('Weights');
  "IW{1,1}(18,:)'" : Constant  Value=[0.1527045320755019142122677067163749597966670989990234375;-0.8117623129171340767840092667029239237308502197265625;-0.36172319163400035169075863450416363775730133056640625;0.3900349947294039498757456385646946728229522705078125;-0.79793631485410987380646474775858223438262939453125;0.418218719424645446469668286226806230843067169189453125;0.1772573155532365107855952146564959548413753509521484375;-0.21746718578422929990523471133201383054256439208984375;-0.39520754370147626044484923113486729562282562255859375;-0.724349725743480998829681993811391294002532958984375;0.69902413536385143988383106261608190834522247314453125;0.85566549609338526938273616906371898949146270751953125]
      mask Display: e = 0.06;c1 = [120 150 230]/255;c2 = ([120 150 230]+0)/383;c3 = ([120 150 230]+128)/383;patch([0 1 1 0],[0 0 1 1],c1);patch([0 1 1 1-e 1-e 0+e],[0 0 1 1-e 0+e 0+e],c2);patch([0 0 1 1-e 0+e 0+e],[0 1 1 1-e 1-e 0+e],c3);plot([0 1 1 0 0],[0 0 1 1 0]);disp('Weights');
  "IW{1,1}(19,:)'" : Constant  Value=[-0.15537764851670987642506815973320044577121734619140625;0.51800555057346542309204551202128641307353973388671875;0.30332757930638909460441254850593395531177520751953125;0.6480405646433691213559313837322406470775604248046875;0.170205250810118002835480410794843919575214385986328125;0.470125897669795123068325892745633609592914581298828125;-0.74806880202543502011991449762717820703983306884765625;-0.380418545647730976799749669226002879440784454345703125;-0.13513979416318633308691232741693966090679168701171875;-0.7444070999112633035821318117086775600910186767578125;-0.56643841111369230834071686331299133598804473876953125;0.7386510425871575247214195769629441201686859130859375]
      mask Display: e = 0.06;c1 = [120 150 230]/255;c2 = ([120 150 230]+0)/383;c3 = ([120 150 230]+128)/383;patch([0 1 1 0],[0 0 1 1],c1);patch([0 1 1 1-e 1-e 0+e],[0 0 1 1-e 0+e 0+e],c2);patch([0 0 1 1-e 0+e 0+e],[0 1 1 1-e 1-e 0+e],c3);plot([0 1 1 0 0],[0 0 1 1 0]);disp('Weights');
  "IW{1,1}(2,:)'" : Constant  Value=[0.8280854681444356213404489608365111052989959716796875;0.50525796687602098078428980443277396261692047119140625;-0.1809179598402941013812750270517426542937755584716796875;-0.02133050340167121083911894174889312125742435455322265625;0.217665307140996799883936319019994698464870452880859375;0.62874784612109679837743669850169681012630462646484375;0.48195855591794500849545102028059773147106170654296875;-0.273842181201820411562408708050497807562351226806640625;-0.280176519180449279389222283498384058475494384765625;0.7217995467128532904865778618841432034969329833984375;-0.1314785261277242323085800990156712941825389862060546875;0.80414994744934442660877493835869245231151580810546875]
      mask Display: e = 0.06;c1 = [120 150 230]/255;c2 = ([120 150 230]+0)/383;c3 = ([120 150 230]+128)/383;patch([0 1 1 0],[0 0 1 1],c1);patch([0 1 1 1-e 1-e 0+e],[0 0 1 1-e 0+e 0+e],c2);patch([0 0 1 1-e 0+e 0+e],[0 1 1 1-e 1-e 0+e],c3);plot([0 1 1 0 0],[0 0 1 1 0]);disp('Weights');
  "IW{1,1}(20,:)'" : Constant  Value=[0.69619064710058486955546186436549760401248931884765625;0.90998481495725080936409767673467285931110382080078125;0.2847856276968201427735039032995700836181640625;-0.0282714066929078446099854460271671996451914310455322265625;-0.00201087137321503441056425032229526550509035587310791015625;-0.09618575766572114160712914099349291063845157623291015625;0.880701914318813283699682870064862072467803955078125;-0.33425085187386505136686309924698434770107269287109375;-0.11549170884861771624319004558856249786913394927978515625;0.82925468127508106253031883170478977262973785400390625;-0.041400638089525328144890892190232989378273487091064453125;0.3779744442410513105556901791715063154697418212890625]
      mask Display: e = 0.06;c1 = [120 150 230]/255;c2 = ([120 150 230]+0)/383;c3 = ([120 150 230]+128)/383;patch([0 1 1 0],[0 0 1 1],c1);patch([0 1 1 1-e 1-e 0+e],[0 0 1 1-e 0+e 0+e],c2);patch([0 0 1 1-e 0+e 0+e],[0 1 1 1-e 1-e 0+e],c3);plot([0 1 1 0 0],[0 0 1 1 0]);disp('Weights');
  "IW{1,1}(3,:)'" : Constant  Value=[-0.11020050081225975235899028348285355605185031890869140625;-0.427242203265760178698684512710315175354480743408203125;0.2589011269406296111839083096128888428211212158203125;-0.279239503366896679725783769754343666136264801025390625;1.0549167804592565200749731957330368459224700927734375;-0.72456741433533877749795237832586281001567840576171875;-0.6094680543584356513520106091164052486419677734375;0.87789144883863878821017578957253135740756988525390625;-0.0532416218343572944515784683972015045583248138427734375;0.2062233955018083209065338223808794282376766204833984375;0.1788974640741682609057505715099978260695934295654296875;-0.152965778847275635232705326416180469095706939697265625]
      mask Display: e = 0.06;c1 = [120 150 230]/255;c2 = ([120 150 230]+0)/383;c3 = ([120 150 230]+128)/383;patch([0 1 1 0],[0 0 1 1],c1);patch([0 1 1 1-e 1-e 0+e],[0 0 1 1-e 0+e 0+e],c2);patch([0 0 1 1-e 0+e 0+e],[0 1 1 1-e 1-e 0+e],c3);plot([0 1 1 0 0],[0 0 1 1 0]);disp('Weights');
  "IW{1,1}(4,:)'" : Constant  Value=[0.1083861867889745755899610912820207886397838592529296875;0.74606772093881013052651951511506922543048858642578125;-0.4374021524445057540475545465596951544284820556640625;0.29386544016977722559857966189156286418437957763671875;0.8281352420645713419133926436188630759716033935546875;-0.494242858286547070978400597596191801130771636962890625;0.5398188747203607196212260532774962484836578369140625;0.2319124475814751951130432416903204284608364105224609375;-0.43419482015553356735182433112640865147113800048828125;0.2059587389162732817826650943970889784395694732666015625;-0.484374157482609091207592655337066389620304107666015625;0.7702788896167189758301674373797141015529632568359375]
      mask Display: e = 0.06;c1 = [120 150 230]/255;c2 = ([120 150 230]+0)/383;c3 = ([120 150 230]+128)/383;patch([0 1 1 0],[0 0 1 1],c1);patch([0 1 1 1-e 1-e 0+e],[0 0 1 1-e 0+e 0+e],c2);patch([0 0 1 1-e 0+e 0+e],[0 1 1 1-e 1-e 0+e],c3);plot([0 1 1 0 0],[0 0 1 1 0]);disp('Weights');
  "IW{1,1}(5,:)'" : Constant  Value=[-0.7016335011871637217240049722022376954555511474609375;-0.498627885122845337928509934499743394553661346435546875;0.25542143157557661847789631792693398892879486083984375;0.10997387592788086807527037080944865010678768157958984375;-0.787294516165899072035472272546030580997467041015625;-0.6178010669914140162717330895247869193553924560546875;0.610034370030688055663858904154039919376373291015625;0.481562581286917590350782347741187550127506256103515625;0.01348282733836262368976033343415110721252858638763427734375;-0.63076358873770355106813667589449323713779449462890625;-0.74804302622691676294408580361050553619861602783203125;-0.082156726830043158571470485185272991657257080078125]
      mask Display: e = 0.06;c1 = [120 150 230]/255;c2 = ([120 150 230]+0)/383;c3 = ([120 150 230]+128)/383;patch([0 1 1 0],[0 0 1 1],c1);patch([0 1 1 1-e 1-e 0+e],[0 0 1 1-e 0+e 0+e],c2);patch([0 0 1 1-e 0+e 0+e],[0 1 1 1-e 1-e 0+e],c3);plot([0 1 1 0 0],[0 0 1 1 0]);disp('Weights');
  "IW{1,1}(6,:)'" : Constant  Value=[0.5243593018463756916247575645684264600276947021484375;-0.67720609986001500946173337069922126829624176025390625;0.8780847264004962848815694087534211575984954833984375;0.0793390762945860583688073575103771872818470001220703125;0.1500447904619488515010061746579594910144805908203125;0.5962839665124242127802745017106644809246063232421875;0.9071326265562602575442952002049423754215240478515625;-0.01132779557878992558739295049008433124981820583343505859375;-0.49849349479581117616788787927362136542797088623046875;-0.15637925153336329486819522571749985218048095703125;0.321341580481250777001633878171560354530811309814453125;-0.4665281414931339298846069141291081905364990234375]
      mask Display: e = 0.06;c1 = [120 150 230]/255;c2 = ([120 150 230]+0)/383;c3 = ([120 150 230]+128)/383;patch([0 1 1 0],[0 0 1 1],c1);patch([0 1 1 1-e 1-e 0+e],[0 0 1 1-e 0+e 0+e],c2);patch([0 0 1 1-e 0+e 0+e],[0 1 1 1-e 1-e 0+e],c3);plot([0 1 1 0 0],[0 0 1 1 0]);disp('Weights');
  "IW{1,1}(7,:)'" : Constant  Value=[0.4279798098204639078545596930780448019504547119140625;-0.59967254725053120711919518726062960922718048095703125;-0.469706736611180897256190291955135762691497802734375;0.45799945084672699646688442953745834529399871826171875;0.459602509513506396476856252775178290903568267822265625;0.471897745050566419511284266263828612864017486572265625;0.7150859720588460533008401398546993732452392578125;-0.62696214320647836171218614254030399024486541748046875;-0.24082786097717756579328352017910219728946685791015625;0.81553908854845513776155030427617020905017852783203125;-0.03253807079923752565431271932538948021829128265380859375;0.54632902575302677572466336641809903085231781005859375]
      mask Display: e = 0.06;c1 = [120 150 230]/255;c2 = ([120 150 230]+0)/383;c3 = ([120 150 230]+128)/383;patch([0 1 1 0],[0 0 1 1],c1);patch([0 1 1 1-e 1-e 0+e],[0 0 1 1-e 0+e 0+e],c2);patch([0 0 1 1-e 0+e 0+e],[0 1 1 1-e 1-e 0+e],c3);plot([0 1 1 0 0],[0 0 1 1 0]);disp('Weights');
  "IW{1,1}(8,:)'" : Constant  Value=[0.12103768379495831453152021595087717287242412567138671875;-0.78731090111940338349683088381425477564334869384765625;0.30839231491739749202452003373764455318450927734375;-0.285233556123715203955981678518583066761493682861328125;-0.81014378243988238725847850218997336924076080322265625;0.89900602150388275735082288520061410963535308837890625;-0.00903590095066473565632580999817946576513350009918212890625;-0.1152466871865962527721194419427774846553802490234375;0.043168544227166684434937593550785095430910587310791015625;-0.6995764213948414411703424775623716413974761962890625;-0.5838131779797353093641731902607716619968414306640625;-0.0370774862742406507987169561602058820426464080810546875]
      mask Display: e = 0.06;c1 = [120 150 230]/255;c2 = ([120 150 230]+0)/383;c3 = ([120 150 230]+128)/383;patch([0 1 1 0],[0 0 1 1],c1);patch([0 1 1 1-e 1-e 0+e],[0 0 1 1-e 0+e 0+e],c2);patch([0 0 1 1-e 0+e 0+e],[0 1 1 1-e 1-e 0+e],c3);plot([0 1 1 0 0],[0 0 1 1 0]);disp('Weights');
  "IW{1,1}(9,:)'" : Constant  Value=[0.401162234370265047278536485464428551495075225830078125;0.50030072449366091991151961337891407310962677001953125;0.2279850905693179274891235763789154589176177978515625;-0.6559591695195743366042506750090979039669036865234375;-0.77832497336603656545861440463340841233730316162109375;-0.59033434188533207009896841555018909275531768798828125;-0.85126215646387304314401944793644361197948455810546875;-0.31850115955207047857555835435050539672374725341796875;0.0036303605183199451345021913084565312601625919342041015625;-0.568104215747422092164242712897248566150665283203125;-0.50821808458320283374831660694326274096965789794921875;-0.11403566068729843741014207125772372819483280181884765625]
      mask Display: e = 0.06;c1 = [120 150 230]/255;c2 = ([120 150 230]+0)/383;c3 = ([120 150 230]+128)/383;patch([0 1 1 0],[0 0 1 1],c1);patch([0 1 1 1-e 1-e 0+e],[0 0 1 1-e 0+e 0+e],c2);patch([0 0 1 1-e 0+e 0+e],[0 1 1 1-e 1-e 0+e],c3);plot([0 1 1 0 0],[0 0 1 1 0]);disp('Weights');
  Mux : Mux  Inputs=20
      mask Display: e = 0.06;c1 = [120 150 230]/255;c2 = ([120 150 230]+0)/383;c3 = ([120 150 230]+128)/383;patch([0 1 1 0],[0 0 1 1],c1);patch([0 1 1 1-e 1-e 0+e],[0 0 1 1-e 0+e 0+e],c2);patch([0 0 1 1-e 0+e 0+e],[0 1 1 1-e 1-e 0+e],c3);plot([0 1 1 0 0],[0 0 1 1 0]);disp('Mux');
  dotprod{1..20} (20 alike) : neural/Weight Functions/dotprod
  "iz{1,1}" : Outport
      mask Display: e = 0.06;c1 = [120 230 180]/255;c2 = ([120 230 180]+0)/(256+128);c3 = ([120 230 180]+128)/(256+128);patch([0 1 1 0],[0 0 1 1],c1);patch([0 1 1 1-e 1-e 0+e],[0 0 1 1-e 0+e 0+e],c2);patch([0 0 1 1-e 0+e 0+e],[0 1 1 1-e 1-e 0+e],c3);plot([0 1 1 0 0],[0 0 1 1 0]);
  wires:
  "IW{1,1}(1,:)'"/1 -> dotprod1/1
  "pd{1,1}"/1 -> dotprod1/2, dotprod2/2, dotprod3/2, dotprod4/2, dotprod5/2, dotprod6/2, dotprod7/2, dotprod8/2, dotprod9/2, dotprod10/2, dotprod11/2, dotprod12/2, dotprod13/2, dotprod14/2, dotprod15/2, dotprod16/2, dotprod17/2, dotprod18/2, dotprod19/2, dotprod20/2
  dotprod1/1 -> Mux/1
  "IW{1,1}(2,:)'"/1 -> dotprod2/1
  dotprod2/1 -> Mux/2
  "IW{1,1}(3,:)'"/1 -> dotprod3/1
  dotprod3/1 -> Mux/3
  "IW{1,1}(4,:)'"/1 -> dotprod4/1
  dotprod4/1 -> Mux/4
  "IW{1,1}(5,:)'"/1 -> dotprod5/1
  dotprod5/1 -> Mux/5
  "IW{1,1}(6,:)'"/1 -> dotprod6/1
  dotprod6/1 -> Mux/6
  "IW{1,1}(7,:)'"/1 -> dotprod7/1
  dotprod7/1 -> Mux/7
  "IW{1,1}(8,:)'"/1 -> dotprod8/1
  dotprod8/1 -> Mux/8
  "IW{1,1}(9,:)'"/1 -> dotprod9/1
  dotprod9/1 -> Mux/9
  "IW{1,1}(10,:)'"/1 -> dotprod10/1
  dotprod10/1 -> Mux/10
  "IW{1,1}(11,:)'"/1 -> dotprod11/1
  dotprod11/1 -> Mux/11
  "IW{1,1}(12,:)'"/1 -> dotprod12/1
  dotprod12/1 -> Mux/12
  "IW{1,1}(13,:)'"/1 -> dotprod13/1
  dotprod13/1 -> Mux/13
  "IW{1,1}(14,:)'"/1 -> dotprod14/1
  dotprod14/1 -> Mux/14
  "IW{1,1}(15,:)'"/1 -> dotprod15/1
  dotprod15/1 -> Mux/15
  "IW{1,1}(16,:)'"/1 -> dotprod16/1
  dotprod16/1 -> Mux/16
  "IW{1,1}(17,:)'"/1 -> dotprod17/1
  dotprod17/1 -> Mux/17
  "IW{1,1}(18,:)'"/1 -> dotprod18/1
  dotprod18/1 -> Mux/18
  "IW{1,1}(19,:)'"/1 -> dotprod19/1
  dotprod19/1 -> Mux/19
  "IW{1,1}(20,:)'"/1 -> dotprod20/1
  dotprod20/1 -> Mux/20
  Mux/1 -> "iz{1,1}"/1

== system clonado_controlador/MLP 20 14400/Function Fitting Neural Network/Layer 2/Delays 1 ==
  "p{2}" : Inport  PortDimensions=20
      mask Display: e = 0.06;c1 = [120 230 180]/255;c2 = ([120 230 180]+0)/(256+128);c3 = ([120 230 180]+128)/(256+128);patch([0 1 1 0],[0 0 1 1],c1);patch([0 1 1 1-e 1-e 0+e],[0 0 1 1-e 0+e 0+e],c2);patch([0 0 1 1-e 0+e 0+e],[0 1 1 1-e 1-e 0+e],c3);plot([0 1 1 0 0],[0 0 1 1 0]);
  mux : Mux  Inputs=1
      mask Display: e = 0.06;c1 = [120 150 230]/255;c2 = ([120 150 230]+0)/383;c3 = ([120 150 230]+128)/383;patch([0 1 1 0],[0 0 1 1],c1);patch([0 1 1 1-e 1-e 0+e],[0 0 1 1-e 0+e 0+e],c2);patch([0 0 1 1-e 0+e 0+e],[0 1 1 1-e 1-e 0+e],c3);plot([0 1 1 0 0],[0 0 1 1 0]);disp('Mux')
  "pd{2,1}" : Outport
      mask Display: e = 0.06;c1 = [120 230 180]/255;c2 = ([120 230 180]+0)/(256+128);c3 = ([120 230 180]+128)/(256+128);patch([0 1 1 0],[0 0 1 1],c1);patch([0 1 1 1-e 1-e 0+e],[0 0 1 1-e 0+e 0+e],c2);patch([0 0 1 1-e 0+e 0+e],[0 1 1 1-e 1-e 0+e],c3);plot([0 1 1 0 0],[0 0 1 1 0]);
  wires:
  "p{2}"/1 -> mux/1
  mux/1 -> "pd{2,1}"/1

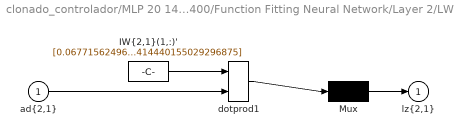
== system clonado_controlador/MLP 20 14400/Function Fitting Neural Network/Layer 2/LW{2,1} ==
  "ad{2,1}" : Inport  PortDimensions=20
      mask Display: e = 0.06;c1 = [120 230 180]/255;c2 = ([120 230 180]+0)/(256+128);c3 = ([120 230 180]+128)/(256+128);patch([0 1 1 0],[0 0 1 1],c1);patch([0 1 1 1-e 1-e 0+e],[0 0 1 1-e 0+e 0+e],c2);patch([0 0 1 1-e 0+e 0+e],[0 1 1 1-e 1-e 0+e],c3);plot([0 1 1 0 0],[0 0 1 1 0]);
  "IW{2,1}(1,:)'" : Constant  Value=[0.0677156249678993182872233091984526254236698150634765625;-0.12228039723860083254347586034782580099999904632568359375;0.2342191697759701540793031426801462657749652862548828125;-0.85567951204279413257580699792015366256237030029296875;-0.38409086445512186092088313671411015093326568603515625;-0.0515139221321740115033804841004894115030765533447265625;-0.812718581292923847314568774891085922718048095703125;1.1966667727687987365925437188707292079925537109375;-0.1377146020325037134579559960911865346133708953857421875;-0.255778556260732869986895821057260036468505859375;0.59200014698152092496030718393740244209766387939453125;0.037579688031091289246443665206243167631328105926513671875;0.24028296485295375095603276349720545113086700439453125;0.50296048223007228106240518172853626310825347900390625;-1.3419519654909635164585779421031475067138671875;0.1670697004417700248790623618333484046161174774169921875;1.0586026605329976746361353434622287750244140625;0.288403742391155348823161830296157859265804290771484375;1.1862702385394545689933920584735460579395294189453125;0.4019777547788041527354607751476578414440155029296875]
      mask Display: e = 0.06;c1 = [120 150 230]/255;c2 = ([120 150 230]+0)/383;c3 = ([120 150 230]+128)/383;patch([0 1 1 0],[0 0 1 1],c1);patch([0 1 1 1-e 1-e 0+e],[0 0 1 1-e 0+e 0+e],c2);patch([0 0 1 1-e 0+e 0+e],[0 1 1 1-e 1-e 0+e],c3);plot([0 1 1 0 0],[0 0 1 1 0]);disp('weights');
  Mux : Mux  Inputs=1
      mask Display: e = 0.06;c1 = [120 150 230]/255;c2 = ([120 150 230]+0)/383;c3 = ([120 150 230]+128)/383;patch([0 1 1 0],[0 0 1 1],c1);patch([0 1 1 1-e 1-e 0+e],[0 0 1 1-e 0+e 0+e],c2);patch([0 0 1 1-e 0+e 0+e],[0 1 1 1-e 1-e 0+e],c3);plot([0 1 1 0 0],[0 0 1 1 0]);disp('Mux');
  dotprod1 : neural/Weight Functions/dotprod
  "lz{2,1}" : Outport
      mask Display: e = 0.06;c1 = [120 230 180]/255;c2 = ([120 230 180]+0)/(256+128);c3 = ([120 230 180]+128)/(256+128);patch([0 1 1 0],[0 0 1 1],c1);patch([0 1 1 1-e 1-e 0+e],[0 0 1 1-e 0+e 0+e],c2);patch([0 0 1 1-e 0+e 0+e],[0 1 1 1-e 1-e 0+e],c3);plot([0 1 1 0 0],[0 0 1 1 0]);
  wires:
  "IW{2,1}(1,:)'"/1 -> dotprod1/1
  "ad{2,1}"/1 -> dotprod1/2
  dotprod1/1 -> Mux/1
  Mux/1 -> "lz{2,1}"/1

== matlab function clonado_controlador/Planta no lineal CL/MATLAB Function ==
  data: h1 input; h2 input; y output; dh1 output; u input; k12 input; k2 input; A1 input; A2 input; dh2 output
function [y, dh1, dh2] = fcn(h1, h2, u, k12, k2, A1, A2)
g = 9.81;

delta_h = max(h1 - h2, 0);

q12 = k12 * sqrt(2 * g * delta_h); % caudal intermedio
q2  = k2  * sqrt(2 * g * max(h2, 0)); % caudal de salida

dh1 = (u - q12) / A1;
dh2 = (q12 - q2) / A2;

y = q2;

%el modelo asume flujo solo en un sentido

%se ignora inversión de flujo

%el sistema es válido para niveles positivos

== matlab function clonado_controlador/Planta no lineal CL1/MATLAB Function ==
  data: h1 input; h2 input; y output; dh1 output; u input; k12 input; k2 input; A1 input; A2 input; dh2 output
function [y, dh1, dh2] = fcn(h1, h2, u, k12, k2, A1, A2)
g = 9.81;

delta_h = max(h1 - h2, 0);

q12 = k12 * sqrt(2 * g * delta_h); % caudal intermedio
q2  = k2  * sqrt(2 * g * max(h2, 0)); % caudal de salida

dh1 = (u - q12) / A1;
dh2 = (q12 - q2) / A2;

y = q2;

%el modelo asume flujo solo en un sentido

%se ignora inversión de flujo

%el sistema es válido para niveles positivos
